simulink model "smallsat_adcs_scaffold"  (R2025b)
settings: Solver=ode113  StartTime=0.0  StopTime=17403  RelTol=1e-10  AbsTol=1e-10
InitFcn:
  | P = smallsat_params; if ~exist('adcsCase', 'var'), adcsCase = 'tumble'; end; ic = initial_state_case(P, adcsCase); bdot = size_bdot(P); pointing = size_pointing(P);
undefined symbols (not defined in the file or in its folder): magnetic_field_eci, quat_to_dcm
settings Model: Creator=USER  LastModifiedBy=USER

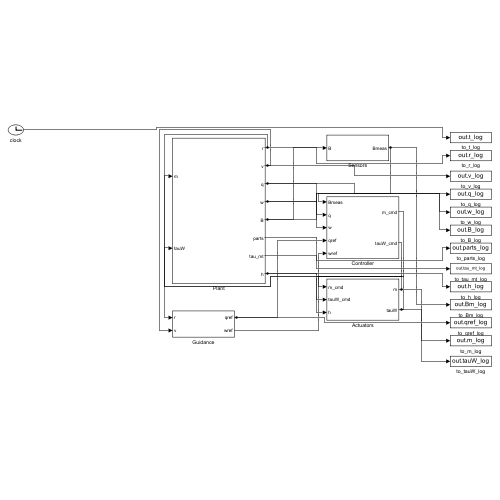
[thumbnail: Simulink's stored preview of the top-level diagram]
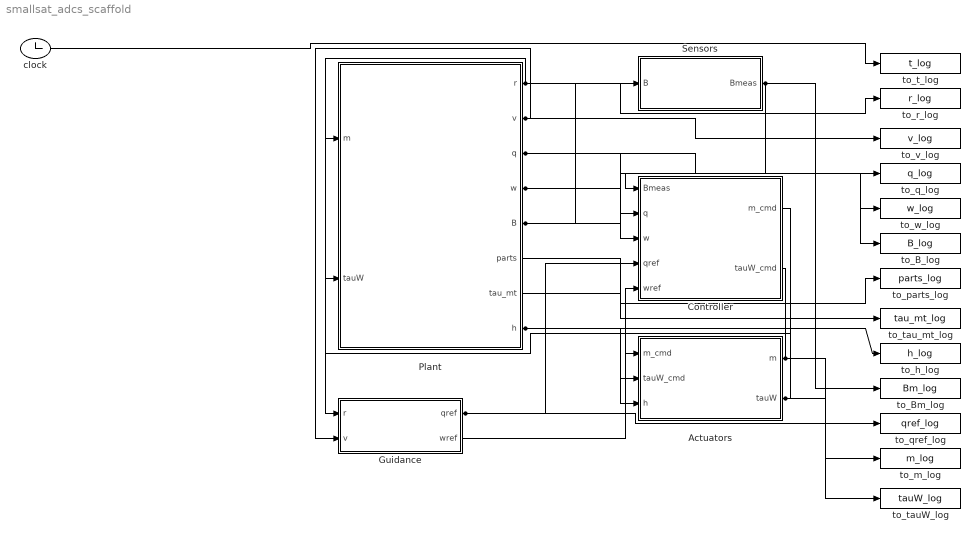
== system smallsat_adcs_scaffold ==
  Actuators : Subsystem
  Controller : Subsystem
  Guidance : Subsystem
  Plant : Subsystem
  Sensors : Subsystem
  clock : Clock
  to_B_log : ToWorkspace  VariableName=B_log  SampleTime=10
  to_Bm_log : ToWorkspace  VariableName=Bm_log  SampleTime=10
  to_h_log : ToWorkspace  VariableName=h_log  SampleTime=10
  to_m_log : ToWorkspace  VariableName=m_log  SampleTime=10
  to_parts_log : ToWorkspace  VariableName=parts_log  SampleTime=10
  to_q_log : ToWorkspace  VariableName=q_log  SampleTime=10
  to_qref_log : ToWorkspace  VariableName=qref_log  SampleTime=10
  to_r_log : ToWorkspace  VariableName=r_log  SampleTime=10
  to_t_log : ToWorkspace  VariableName=t_log  SampleTime=10
  to_tauW_log : ToWorkspace  VariableName=tauW_log  SampleTime=10
  to_tau_mt_log : ToWorkspace  VariableName=tau_mt_log  SampleTime=10
  to_v_log : ToWorkspace  VariableName=v_log  SampleTime=10
  to_w_log : ToWorkspace  VariableName=w_log  SampleTime=10
  wires:
  Plant/5(B) -> Sensors/1(B), to_B_log/1
  Plant/1(r) -> Guidance/1(r), to_r_log/1
  Plant/2(v) -> Guidance/2(v), to_v_log/1
  Sensors/1(Bmeas) -> Controller/1(Bmeas), to_Bm_log/1
  Plant/3(q) -> Controller/2(q), to_q_log/1
  Plant/4(w) -> Controller/3(w), to_w_log/1
  Guidance/1(qref) -> Controller/4(qref), to_qref_log/1
  Guidance/2(wref) -> Controller/5(wref)
  Controller/1(m_cmd) -> Actuators/1(m_cmd)
  Controller/2(tauW_cmd) -> Actuators/2(tauW_cmd)
  Plant/8(h) -> Actuators/3(h), to_h_log/1
  Actuators/1(m) -> Plant/1(m), to_m_log/1
  Actuators/2(tauW) -> Plant/2(tauW), to_tauW_log/1
  clock/1 -> to_t_log/1
  Plant/6(parts) -> to_parts_log/1
  Plant/7(tau_mt) -> to_tau_mt_log/1

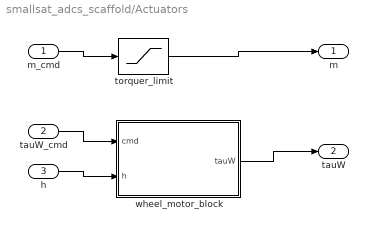
== system smallsat_adcs_scaffold/Actuators ==
  m_cmd : Inport
  tauW_cmd : Inport  Port=2
  h : Inport  Port=3
  torquer_limit : Saturate  UpperLimit=P.mtqMax  LowerLimit=-P.mtqMax
  wheel_motor_block : MATLAB Function  TreatAsAtomicUnit=on
  m : Outport
  tauW : Outport  Port=2
  wires:
  m_cmd/1 -> torquer_limit/1
  torquer_limit/1 -> m/1
  tauW_cmd/1 -> wheel_motor_block/1(cmd)
  h/1 -> wheel_motor_block/2(h)
  wheel_motor_block/1(tauW) -> tauW/1

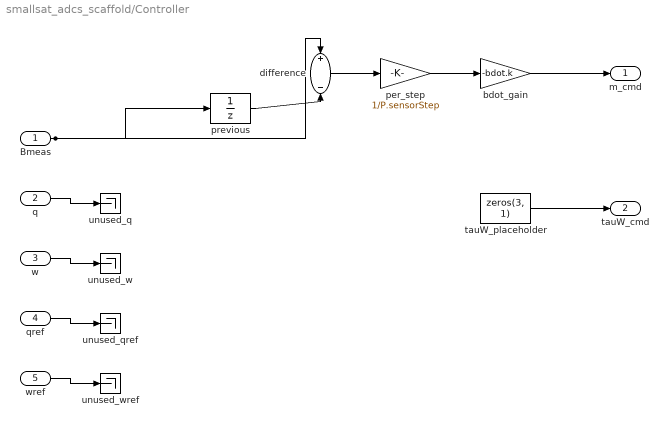
== system smallsat_adcs_scaffold/Controller ==
  Bmeas : Inport
  q : Inport  Port=2
  w : Inport  Port=3
  qref : Inport  Port=4
  wref : Inport  Port=5
  bdot_gain : Gain  Gain=-bdot.k
  difference : Sum  Inputs=+-
  per_step : Gain  Gain=1/P.sensorStep
  previous : UnitDelay  InitialCondition=quat_to_dcm(ic.q)*magnetic_field_eci(ic.r, 0, P)  SampleTime=P.sensorStep  HasFrameUpgradeWarning=on
  tauW_placeholder : Constant  Value=zeros(3, 1)  VectorParams1D=off
  unused_q : Terminator
  unused_qref : Terminator
  unused_w : Terminator
  unused_wref : Terminator
  m_cmd : Outport
  tauW_cmd : Outport  Port=2
  wires:
  q/1 -> unused_q/1
  w/1 -> unused_w/1
  qref/1 -> unused_qref/1
  wref/1 -> unused_wref/1
  Bmeas/1 -> difference/1, previous/1
  previous/1 -> difference/2
  difference/1 -> per_step/1
  per_step/1 -> bdot_gain/1
  bdot_gain/1 -> m_cmd/1
  tauW_placeholder/1 -> tauW_cmd/1

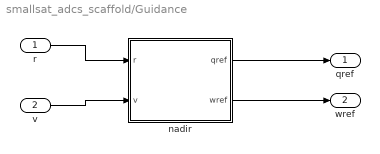
== system smallsat_adcs_scaffold/Guidance ==
  r : Inport
  v : Inport  Port=2
  nadir : MATLAB Function  TreatAsAtomicUnit=on
  qref : Outport
  wref : Outport  Port=2
  wires:
  r/1 -> nadir/1(r)
  v/1 -> nadir/2(v)
  nadir/1(qref) -> qref/1
  nadir/2(wref) -> wref/1

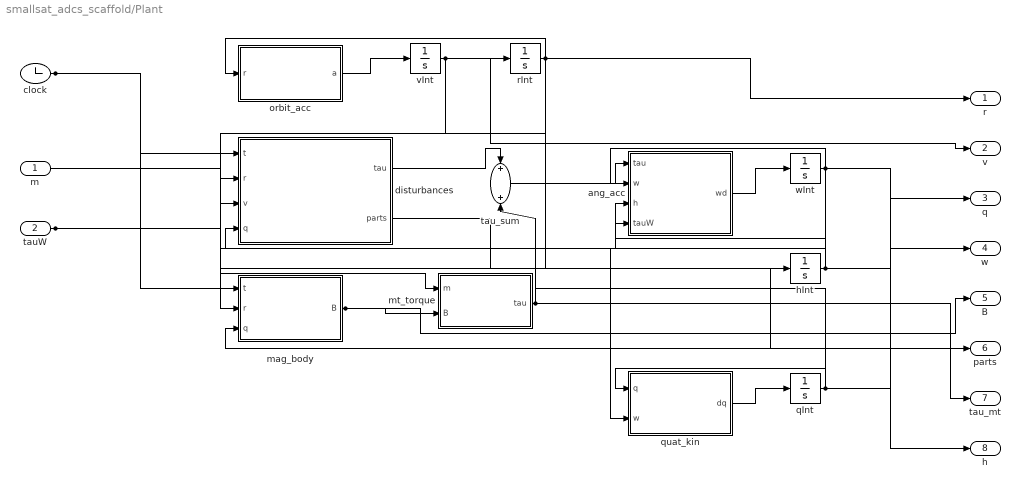
== system smallsat_adcs_scaffold/Plant ==
  m : Inport
  tauW : Inport  Port=2
  ang_acc : MATLAB Function  TreatAsAtomicUnit=on
  clock : Clock
  disturbances : MATLAB Function  TreatAsAtomicUnit=on
  hInt : Integrator  InitialCondition=ic.h
  mag_body : MATLAB Function  TreatAsAtomicUnit=on
  mt_torque : MATLAB Function  TreatAsAtomicUnit=on
  orbit_acc : MATLAB Function  TreatAsAtomicUnit=on
  qInt : Integrator  InitialCondition=ic.q
  quat_kin : MATLAB Function  TreatAsAtomicUnit=on
  rInt : Integrator  InitialCondition=ic.r
  tau_sum : Sum
  vInt : Integrator  InitialCondition=ic.v
  wInt : Integrator  InitialCondition=ic.w
  r : Outport
  v : Outport  Port=2
  q : Outport  Port=3
  w : Outport  Port=4
  B : Outport  Port=5
  parts : Outport  Port=6
  tau_mt : Outport  Port=7
  h : Outport  Port=8
  wires:
  rInt/1 -> orbit_acc/1(r), disturbances/2(r), mag_body/2(r), r/1
  orbit_acc/1(a) -> vInt/1
  vInt/1 -> rInt/1, disturbances/3(v), v/1
  clock/1 -> disturbances/1(t), mag_body/1(t)
  qInt/1 -> disturbances/4(q), mag_body/3(q), quat_kin/1(q), q/1
  m/1 -> mt_torque/1(m)
  mag_body/1(B) -> mt_torque/2(B), B/1
  disturbances/1(tau) -> tau_sum/1
  mt_torque/1(tau) -> tau_sum/2, tau_mt/1
  tau_sum/1 -> ang_acc/1(tau)
  wInt/1 -> ang_acc/2(w), quat_kin/2(w), w/1
  hInt/1 -> ang_acc/3(h), h/1
  tauW/1 -> ang_acc/4(tauW), hInt/1
  ang_acc/1(wd) -> wInt/1
  quat_kin/1(dq) -> qInt/1
  disturbances/2(parts) -> parts/1

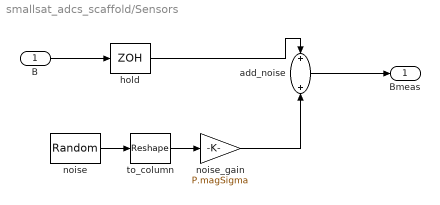
== system smallsat_adcs_scaffold/Sensors ==
  B : Inport
  add_noise : Sum
  hold : ZeroOrderHold  SampleTime=P.sensorStep
  noise : RandomNumber  Seed=[11 22 33]  SampleTime=P.sensorStep
  noise_gain : Gain  Gain=P.magSigma
  to_column : Reshape  OutputDimensionality=Customize  OutputDimensions=[3 1]
  Bmeas : Outport
  wires:
  B/1 -> hold/1
  hold/1 -> add_noise/1
  noise/1 -> to_column/1
  to_column/1 -> noise_gain/1
  noise_gain/1 -> add_noise/2
  add_noise/1 -> Bmeas/1

== matlab function smallsat_adcs_scaffold/Plant/disturbances ==
  data: t input; tau output; r input; v input; q input; parts output; P parameter
function [tau, parts] = disturbances(t, r, v, q, P)
%#codegen
[tau, parts] = disturbance_block(t, r, v, q, P);
end

== matlab function smallsat_adcs_scaffold/Plant/orbit_acc ==
  data: r input; a output; P parameter
function a = orbit_acc(r, P)
%#codegen
a = j2_accel(r, P);
end

== matlab function smallsat_adcs_scaffold/Plant/mag_body ==
  data: t input; B output; r input; q input; P parameter
function B = mag_body(t, r, q, P)
%#codegen
B = quat_to_dcm(q)*magnetic_field_eci(r, t, P);
end

== matlab function smallsat_adcs_scaffold/Plant/mt_torque ==
  data: m input; tau output; B input
function tau = mt_torque(m, B)
%#codegen
tau = cross(m, B);
end

== matlab function smallsat_adcs_scaffold/Plant/ang_acc ==
  data: tau input; wd output; w input; h input; tauW input; P parameter
function wd = ang_acc(tau, w, h, tauW, P)
%#codegen
wd = angular_accel(w, h, tau, tauW, P.inertia);
end

== matlab function smallsat_adcs_scaffold/Plant/quat_kin ==
  data: q input; dq output; w input
function dq = quat_kin(q, w)
%#codegen
dq = quat_rate(q, w);
end

== matlab function smallsat_adcs_scaffold/Guidance/nadir ==
  data: r input; qref output; v input; wref output
function [qref, wref] = nadir(r, v)
%#codegen
[qref, wref] = nadir_reference(r, v);
end

== matlab function smallsat_adcs_scaffold/Actuators/wheel_motor_block ==
  data: cmd input; tauW output; h input; P parameter
function tauW = wheel_motor_block(cmd, h, P)
%#codegen
tauW = wheel_motor(cmd, h, P);
end
